simulink model "EE463_SoftwareProject2_q1_Singlephasecontrolledrectifier"  (R2017b)
settings: Solver=VariableStepDiscrete  StartTime=0.0  StopTime=2.0  MaxStep=1e-4  RelTol=1e-3
libraries: powerlib x23
settings Model: Creator=SiF  LastModifiedBy=SiF

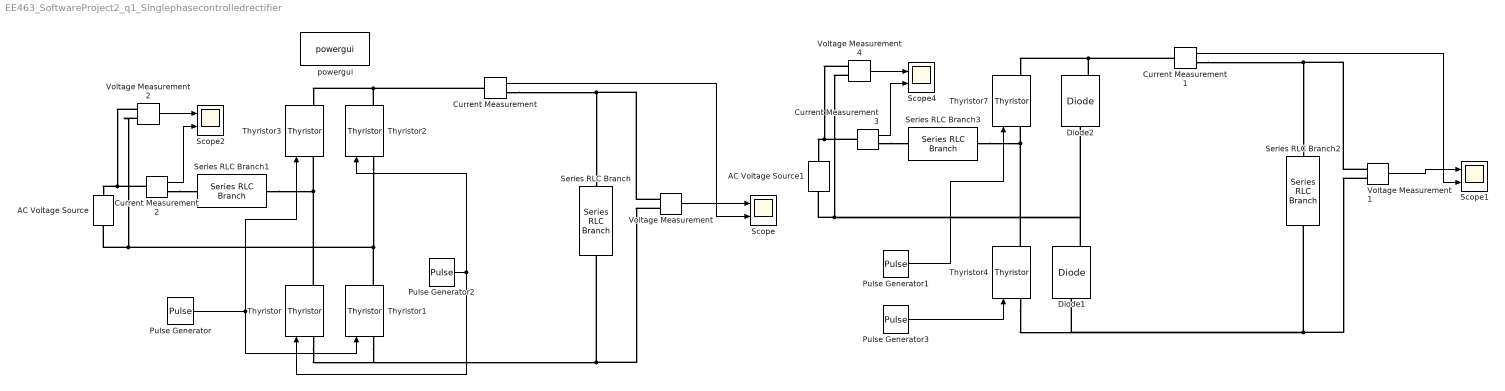
== system EE463_SoftwareProject2_q1_Singlephasecontrolledrectifier ==
  AC Voltage Source : powerlib/Electrical Sources/AC Voltage Source  Amplitude=325.26  Phase=0  Frequency=50  SampleTime=1e-6  Measurements=None  BusType=swing  Pref=10e3  Qref=0  Qmin=-inf  Qmax=+inf
  AC Voltage Source1 : powerlib/Electrical Sources/AC Voltage Source  Amplitude=325.26  Phase=0  Frequency=50  SampleTime=1e-6  Measurements=None  BusType=swing  Pref=10e3  Qref=0  Qmin=-inf  Qmax=+inf
  Current Measurement{,1..3} (4 alike) : powerlib/Measurements/Current Measurement  PhasorSimulation=off  OutputType=Complex  PSBequivalent=0
  Diode1 : powerlib/Power Electronics/Diode  Ron=0.001  Lon=0  Vf=0  IC=0  UseSnubber=0  Rs=500  Cs=250e-9  Measurements=on
  Diode2 : powerlib/Power Electronics/Diode  Ron=0.001  Lon=0  Vf=0  IC=0  UseSnubber=0  Rs=500  Cs=250e-9  Measurements=on
  Pulse Generator : DiscretePulseGenerator  PulseType=Time based  Amplitude=3  Period=0.02  PhaseDelay=0.02/360*37
  Pulse Generator1 : DiscretePulseGenerator  PulseType=Time based  Amplitude=3  Period=0.02  PhaseDelay=0.02/360*55
  Pulse Generator2 : DiscretePulseGenerator  PulseType=Time based  Amplitude=3  Period=0.02  PhaseDelay=0.02/360*37+0.01
  Pulse Generator3 : DiscretePulseGenerator  PulseType=Time based  Amplitude=3  Period=0.02  PhaseDelay=0.02/360*55+0.01
  Scope{,1..2,4} (4 alike) : Scope  NumInputPorts=2
  Series RLC Branch : powerlib/Elements/Series RLC Branch  LConnTagsString=__new0  RConnTagsString=__new0  BranchType=RL  Resistance=4  Inductance=200e-3  SetiL0=off  InitialCurrent=0  Capacitance=1e-6  Setx0=off  InitialVoltage=0  Measurements=None
  Series RLC Branch1 : powerlib/Elements/Series RLC Branch  LConnTagsString=__new0  RConnTagsString=__new0  BranchType=L  Resistance=100  Inductance=0.5e-3  SetiL0=off  InitialCurrent=0  Capacitance=1e-6  Setx0=off  InitialVoltage=0  Measurements=None
  Series RLC Branch2 : powerlib/Elements/Series RLC Branch  LConnTagsString=__new0  RConnTagsString=__new0  BranchType=RL  Resistance=4  Inductance=200e-3  SetiL0=off  InitialCurrent=0  Capacitance=1e-6  Setx0=off  InitialVoltage=0  Measurements=None
  Series RLC Branch3 : powerlib/Elements/Series RLC Branch  LConnTagsString=__new0  RConnTagsString=__new0  BranchType=L  Resistance=100  Inductance=0.5e-3  SetiL0=off  InitialCurrent=0  Capacitance=1e-6  Setx0=off  InitialVoltage=0  Measurements=None
  Thyristor{,1..4,7} (6 alike) : powerlib/Power Electronics/Thyristor  Ron=0.001  Lon=0  Vf=0  IC=0  Rs=500  Cs=250e-9  Measurements=on
  Voltage Measurement{,1..2,4} (4 alike) : powerlib/Measurements/Voltage Measurement  PhasorSimulation=off  OutputType=Complex  PSBequivalent=0
  powergui : powerlib/powergui  Priority=1  SimulationMode=Discrete  SampleTime=1e-6  frequency=60  Iterations=50  frequencyindice=50  Pbase=100e6  ErrMax=1e-4  UnitsV=kV  UnitsW=MW  buscounter=0  FunctionMessages=off  echomessages=off  EnableUseOfTLC=off  CurrentSourceSwitches=off  DisableSnubberDevices=off  DisableRonSwitches=off  DisableVfSwitches=off  DisplayEquations=off  SolverType=Tustin/Backward Euler (TBE)  Interpol=off  ExternalGateDelay=off  methode=off  Ts=100  x0status=blocks  SPID=on  SwTol=0  HookPort=off  RestoreLinks=warning  ResistiveCurrentMeasurement=off  Frange=[0:2:500]  Ylog=off  Xlog=on  ShowGrid=off  save=off  variable=ZData  structure=0  ZoomFFT=off  StartTime=0.0  cycles=1  DisplayStyle=1  fundamental=60  FreqAxis=off  MaxFrequency=1000  frequencyindicesteady=1  RmsSteady=1  display=off
  wires:
  Voltage Measurement1/1 -> Scope1/1
  Pulse Generator/1 -> Thyristor3/1, Thyristor1/1
  Pulse Generator1/1 -> Thyristor7/1
  Voltage Measurement/1 -> Scope/1
  Pulse Generator2/1 -> Thyristor/1, Thyristor2/1
  Current Measurement/1 -> Scope/2
  Pulse Generator3/1 -> Thyristor4/1
  Current Measurement1/1 -> Scope1/2
  Voltage Measurement2/1 -> Scope2/1
  Current Measurement2/1 -> Scope2/2
  Current Measurement3/1 -> Scope4/2
  Voltage Measurement4/1 -> Scope4/1
  connections:
  Voltage Measurement/LConn1 -- Current Measurement/RConn1 -- Series RLC Branch/LConn1
  Voltage Measurement/LConn2 -- Series RLC Branch/RConn1 -- Thyristor/LConn1 -- Thyristor1/LConn1
  Thyristor/RConn1 -- Series RLC Branch1/LConn1 -- Thyristor3/LConn1
  Thyristor2/LConn1 -- Thyristor1/RConn1 -- Voltage Measurement2/LConn2 -- AC Voltage Source/LConn1
  Diode2/LConn1 -- Diode1/RConn1 -- Voltage Measurement4/LConn2 -- AC Voltage Source1/LConn1
  Voltage Measurement1/LConn2 -- Thyristor4/LConn1 -- Diode1/LConn1 -- Series RLC Branch2/RConn1
  Diode2/RConn1 -- Current Measurement1/LConn1 -- Thyristor7/RConn1
  Series RLC Branch3/LConn1 -- Thyristor4/RConn1 -- Thyristor7/LConn1
  Thyristor2/RConn1 -- Current Measurement/LConn1 -- Thyristor3/RConn1
  Voltage Measurement1/LConn1 -- Current Measurement1/RConn1 -- Series RLC Branch2/LConn1
  Current Measurement2/RConn1 -- Series RLC Branch1/RConn1
  Current Measurement2/LConn1 -- Voltage Measurement2/LConn1 -- AC Voltage Source/RConn1
  Current Measurement3/RConn1 -- Series RLC Branch3/RConn1
  Current Measurement3/LConn1 -- Voltage Measurement4/LConn1 -- AC Voltage Source1/RConn1
